simulink model "system"  (R2023b)
settings: Solver=VariableStepAuto  StartTime=0.0  StopTime=10.0  RelTol=1e-3
values from neighbouring files (symbols this model uses):
  den = [1 (R1*C1+R2*C2+R1*C2)/(R1*R2*C1*C2) 1/(R1*R2*C1*C2)]    [controlled_system.m]
  num = 1/(R1*R2*C1*C2)    (= 20.6611570248)    [controlled_system.m]
undefined symbols (not defined in the file or in its folder): DiscIntNeverNeededParam
settings Model: Creator=Administrator  LastModifiedBy=Administrator

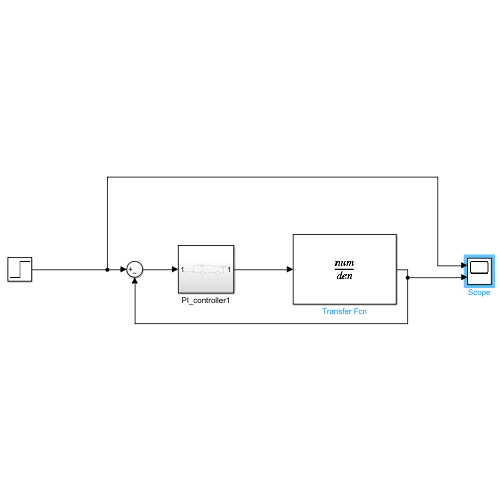
[thumbnail: Simulink's stored preview of the top-level diagram]
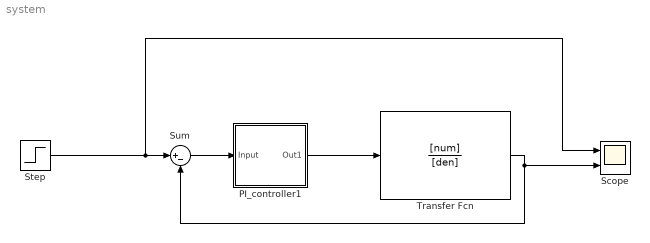
== system system ==
  PI_controller1 : Subsystem
  Scope : Scope  NumInputPorts=2
  Step : Step  SampleTime=0
  Sum : Sum  Inputs=|+-
  Transfer Fcn : TransferFcn  Numerator=[num]  Denominator=[den]
  wires:
  Step/1 -> Scope/1, Sum/1
  Transfer Fcn/1 -> Sum/2, Scope/2
  Sum/1 -> PI_controller1/1(Input)
  PI_controller1/1(Out1) -> Transfer Fcn/1

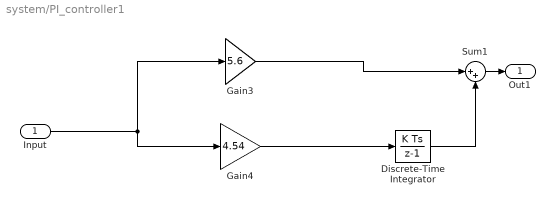
== system system/PI_controller1 ==
  Input : Inport
  Discrete-Time Integrator : DiscreteIntegrator  SampleTime=-1  ICPrevOutput=DiscIntNeverNeededParam  ICPrevScaledInput=DiscIntNeverNeededParam
  Gain3 : Gain  Gain=5.6
  Gain4 : Gain  Gain=4.54
  Sum1 : Sum  Inputs=|++
  Out1 : Outport
  wires:
  Gain4/1 -> Discrete-Time Integrator/1
  Discrete-Time Integrator/1 -> Sum1/2
  Gain3/1 -> Sum1/1
  Sum1/1 -> Out1/1
  Input/1 -> Gain3/1, Gain4/1
